simulink model "SiL_gram"  (R2025b)
settings: Solver=ode2  StartTime=0.0  StopTime=t_end  FixedStep=1/400  RelTol=1e-3
PreLoadFcn:
  | stepsize_sim = evalin('base', get_param(bdroot, 'FixedStep'));
undefined symbols (not defined in the file or in its folder): defaultConsts, defaultWP, DiscIntNeverNeededParam, dspblkCoreblockFVToolHelper, gcbh, navConsts, sensors, stepsize_ctrl
libraries: simulink x7, sharedutil x1, sharedtransform x1, aerolibanimutils x1
(part 1 of 3)
settings Model: Creator=ac112430  LastModifiedBy=ac124458
settings SolverCC: AlgebraicLoopSolver=TrustRegion
settings OptimizationCC: DefaultParameterBehavior=Inlined  DefaultUnderspecifiedDataType=single  ReuseModelBlockBuffer=off  PassReuseOutputArgsAs=Individual arguments  EfficientTunableParamExpr=on
settings DebuggingCC: ParameterPrecisionLossMsg=none  ParameterTunabilityLossMsg=error  UnconnectedInputMsg=warning  UnconnectedOutputMsg=warning  UnconnectedLineMsg=warning  ArithmeticOperatorsInVariantConditions=warning
settings HardwareCC: ProdBitPerPointer=32.0  ProdBitPerSizeT=32.0  ProdBitPerPtrDiffT=32.0  ProdLargestAtomicInteger=Long  ProdLargestAtomicFloat=Double  ProdIntDivRoundTo=Undefined  ProdWordSize=32.0  ProdHWDeviceType=ARM Compatible->ARM Cortex
settings ModelReferenceCC: EnableRefExpFcnMdlSchedulingChecks=on  ModelReferenceNumInstancesAllowed=Single  ModelReferenceMinAlgLoopOccurrences=on  PropagateSignalLabelsOutOfModel=off
settings SFSimCC: SimUseLocalCustomCode=off  MATLABDynamicMemAlloc=off  CustomCodeUndefinedFunction=UseInterfaceOnly
settings RTWCC: SystemTargetFile=ert.tlc  GenCodeOnly=on  TemplateMakefile=ert_default_tmf  RTWUseLocalCustomCode=off  IncludeHyperlinkInReport=on  GPUComputeCapability=3.5  Description=Embedded Coder
settings CodeAppCC: IgnoreCustomStorageClasses=off  StateflowObjectComments=on
settings ERTTargetCC: ERTCustomFileTemplate=example_file_process.tlc  ConvertIfToSwitch=off  SuppressUnreachableDefaultCases=off  DynamicArrayContainerType=coder::array  TargetLangStandard=C99 (ISO)  GenerateSampleERTMain=on  SupportComplex=off

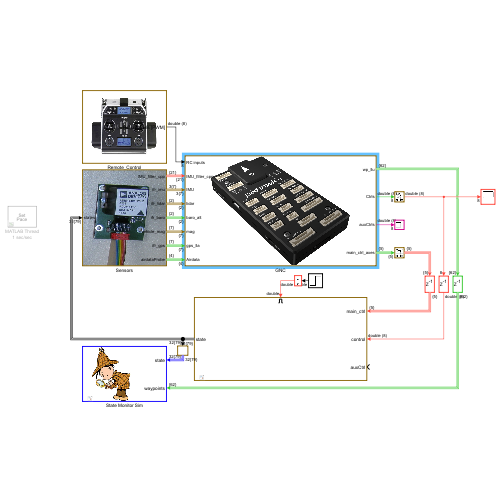
[thumbnail: Simulink's stored preview of the top-level diagram]
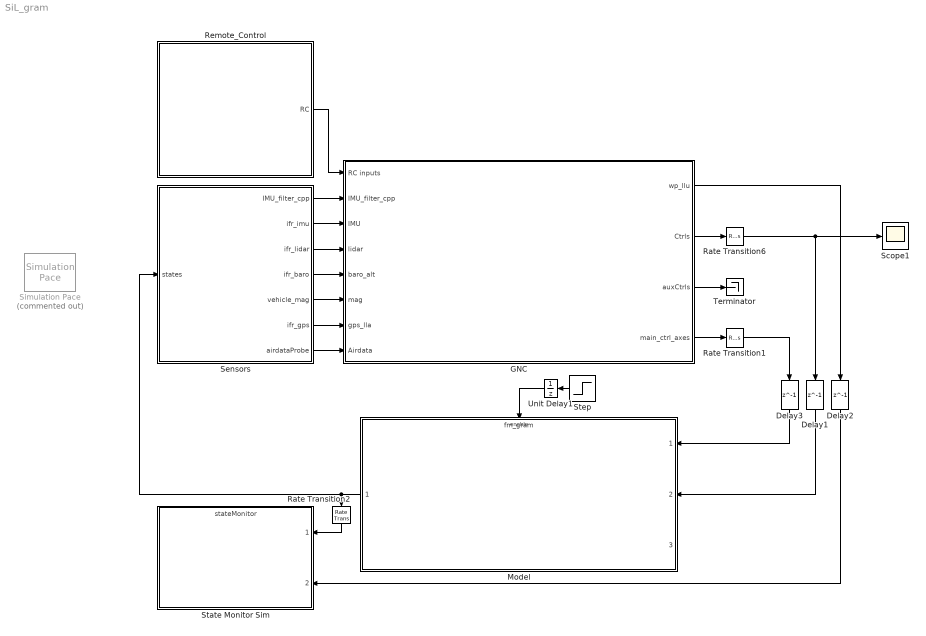
== system SiL_gram ==
  Delay1 : Delay  DelayLength=1  InitialCondition=0
  Delay2 : Delay  DelayLength=1  InitialCondition=0
  Delay3 : Delay  DelayLength=1  InitialCondition=0
  GNC : Subsystem
      mask Display:
      | image('figures/pixhawk2.png');
      | 
      | %port_label('input', 1, 'RC inputs');
      | %port_label('input', 2, 'IMU');
      | %port_label('input', 3, 'Optical Flow');
      | %port_label('input', 4, 'Sonar');
      | %port_label('input', 5, 'Barometer');
      | %port_label('input', 6, 'Magetometer');
      | %port_label('input', 7, 'GPS');
      | %port_label('input', 8, 'Airdata Probe');
      | 
      | %port_label('output', 1, 'Modes');
      | %port_label('output', 2, 'Warning ID');
      | %port_label('output', 3, 'State monitor data');
      | %port_label('output', 4, '(\delta \xi \eta \zeta \xi2 TW)^T', 'texmode', 'on');
      | %port_label('output', 5, 'Auxiliary controls', 'texmode', 'on');
      | %port_label('output', 6, '(x y z)_{ned}^T', 'texmode', 'on');
      | %port_label('output', 7, '(q1 q2 q3 q4)^T', 'texmode', 'on');
      | %port_label('output', 8, '(v_x v_y v_z)_{ned}^T', 'texmode', 'on');
      | %port_label('output', 9, '(v_{w,x} v_{w,y} v_{w,z})^T', 'texmode', 'on');
  Model : ModelReference  ModelNameDialog=fm_gram.slx  SimulationMode=Normal  ModelReferenceVersion=12.108  EnablePortName=Enable  EnablePortStatesWhenEnabling=held
      mask Display: %image('Library\figures\gram.jpg');
  Rate Transition1 : RateTransition  OutPortSampleTime=stepsize_sim
  Rate Transition2 : RateTransition  OutPortSampleTime=stepsize_mon
  Rate Transition6 : RateTransition  OutPortSampleTime=stepsize_sim
  Remote_Control : Subsystem
      mask Display:
      | image('figures/rc.png');
      | 
      | port_label('output', 1, 'RC channels [PWM]');
  Scope1 : Scope
      settings: ActiveDisplayYMinimum=-1.25  ActiveDisplayYMaximum=1.25
  Sensors : Subsystem
      mask Display:
      | image('figures/Sensoren.jpg');
      | 
      | %port_label('input', 1, 'State');
      | 
      | %port_label('output', 1, 'IMU');
      | %port_label('output', 2, 'Optical Flow');
      | %port_label('output', 3, 'Sonar');
      | %port_label('output', 4, 'Barometer');
      | %port_label('output', 5, 'Magnetometer');
      | %port_label('output', 6, 'GPS');
      | %port_label('output', 7, 'Airdata Probe');
  Simulation Pace : aerolibanimutils/Simulation Pace  Commented=on  SimulationPace=1  SleepMode=MATLAB Thread  OutputPaceError=off  SampleTime=-1
  State Monitor Sim : ModelReference  ModelNameDialog=stateMonitor.slx  SimulationMode=Normal  ModelReferenceVersion=12.19
      mask Display:
      | image('figures/detektiv2.png');
      | 
      | %port_label('input', 1, 'State');
      | %port_label('input', 2, 'V_{wind}','texmode','on');
      | %port_label('input', 3, 'State monitor data');
  Step : Step  Time=defaultConsts.forcesSuppressedTime  SampleTime=0
  Terminator : Terminator
  Unit Delay1 : UnitDelay  InitialCondition=1  SampleTime=-1  HasFrameUpgradeWarning=on
  wires:
  Sensors/2(ifr_imu) -> GNC/3(IMU)
  Sensors/3(ifr_lidar) -> GNC/4(lidar)
  Sensors/4(ifr_baro) -> GNC/5(baro_alt)
  Sensors/5(vehicle_mag) -> GNC/6(mag)
  Sensors/6(ifr_gps) -> GNC/7(gps_lla)
  Sensors/7(airdataProbe) -> GNC/8(Airdata)
  Remote_Control/1(RC) -> GNC/1(RC inputs)
  GNC/2(Ctrls) -> Rate Transition6/1
  GNC/1(wp_llu) -> Delay2/1
  Delay1/1 -> Model/2
  Model/1 -> Sensors/1(states), Rate Transition2/1
  Rate Transition2/1 -> State Monitor Sim/1
  Rate Transition6/1 -> Scope1/1, Delay1/1
  Sensors/1(IMU_filter_cpp) -> GNC/2(IMU_filter_cpp)
  Step/1 -> Unit Delay1/1
  Unit Delay1/1 -> Model/Enable
  Delay2/1 -> State Monitor Sim/2
  GNC/3(auxCtrls) -> Terminator/1
  GNC/4(main_ctrl_axes) -> Rate Transition1/1
  Delay3/1 -> Model/1
  Rate Transition1/1 -> Delay3/1

== system SiL_gram/GNC ==
  RC inputs : Inport
  IMU_filter_cpp : Inport  Port=2  OutDataTypeStr=Bus: ifr_imu_filtered_bus
  IMU : Inport  Port=3  OutDataTypeStr=Bus: ifr_imu
  lidar : Inport  Port=4  OutDataTypeStr=Bus: ifr_lidar
  baro_alt : Inport  Port=5  OutDataTypeStr=Bus: ifr_baro
  mag : Inport  Port=6  OutDataTypeStr=Bus: vehicle_magnetometer_bus
  gps_lla : Inport  Port=7  OutDataTypeStr=Bus: ifr_gps
  Airdata : Inport  Port=8  OutDataTypeStr=Bus: ifr_airdata
  EKF2_emulation : Subsystem
  Guidance_Control : Subsystem
  Postprocessing : Subsystem
  Unit Delay : UnitDelay  SampleTime=-1  HasFrameUpgradeWarning=on
  mavlink_receiver.cpp : Subsystem
  state_estimation : Subsystem
      settings: PortSchema="{\"entries\":[{\"content\":{\"sides\":[{\"content\":{\"connectorIds\":[\"In1\",\"In2\",\"In3\",\"In4\",\"In5\",\"In6\",\"In7\",\"In8\",\"In9\",\"In10\"]},\"type\":\"ConnectorPlacement.EquallySpacedRectSide\",\"uuid\":\"f704c686-db51-4285-959d-e889b94520cd\"},{\"content\":{\"connectorIds\":[\"Out1\",\"Out2\",\"Out3\",\"Out4\",\"Out5\",\"Out6\"],\"side\":\"RIGHT\"},\"type\":\"ConnectorPlacement.EquallySpacedRectSide\",\"uuid\":\"07b64360-9707-41f4-adee-da3792a52092\"},{\"content\":{\"connectorIds\":[\"In11\"],\"side\":\"TOP\"},\"type\":\"ConnectorPlacement.EquallySpacedRectSide\",\"uuid\":\"2f5e8d8a-3f45-40ad-b8f5-d38ec2cbea29\"}]},\"type\":\"ConnectorPlacement.EquallySpacedConnector\",\"uuid\":\"8dcdc60e-7634-4563-a6f8-beae9412036b\"}],\"packageUris\":[\"http://schema.mathworks.com/mf0/Connector/R2020b\"],\"version\":\"1.0\"}"
  wp_llu : Outport  OutDataTypeStr=Bus: waypoint_list_bus
  Ctrls : Outport  Port=2
  auxCtrls : Outport  Port=3
  main_ctrl_axes : Outport  Port=4  OutDataTypeStr=Bus: main_ctrl_axes_bus
  wires:
  Postprocessing/1(Ctrls) -> Ctrls/1
  RC inputs/1 -> mavlink_receiver.cpp/1(inputRC)
  IMU/1 -> mavlink_receiver.cpp/2(IMU)
  lidar/1 -> mavlink_receiver.cpp/3(lidar)
  baro_alt/1 -> mavlink_receiver.cpp/4(baro_alt)
  mag/1 -> mavlink_receiver.cpp/5(mag)
  gps_lla/1 -> mavlink_receiver.cpp/6(gps)
  Airdata/1 -> mavlink_receiver.cpp/7(Airdata)
  mavlink_receiver.cpp/9(RC channels) -> state_estimation/10(RC channels), Guidance_Control/12(RC channels)
  mavlink_receiver.cpp/1(Armed) -> state_estimation/2(armed)
  Guidance_Control/2(controls_0) -> Postprocessing/1(controls_0)
  mavlink_receiver.cpp/2(Time) -> state_estimation/3(clock)
  mavlink_receiver.cpp/3(Gyro) -> EKF2_emulation/2(gyro), state_estimation/4(gyro)
  mavlink_receiver.cpp/8(Accel) -> state_estimation/9(accel), EKF2_emulation/6(accel), Guidance_Control/11(sensor_accel)
  mavlink_receiver.cpp/4(baro) -> EKF2_emulation/3(baro), state_estimation/5(baro)
  mavlink_receiver.cpp/5(magmeter) -> EKF2_emulation/4(mag), state_estimation/6(mag)
  mavlink_receiver.cpp/6(gps_lla) -> EKF2_emulation/5(gps), state_estimation/7(gps)
  mavlink_receiver.cpp/7(status) -> state_estimation/8(status)
  state_estimation/1(time) -> Guidance_Control/2(clock)
  mavlink_receiver.cpp/10(waypoints) -> wp_llu/1, Guidance_Control/13(waypoint_list)
  Postprocessing/2(auxCtrls) -> auxCtrls/1
  Guidance_Control/3(controls_1) -> Postprocessing/2(controls_1)
  state_estimation/5(ac_state) -> Guidance_Control/6(ac_state)
  Unit Delay/1 -> state_estimation/11(main_ctrl_axes)
  state_estimation/3(act_limits) -> Guidance_Control/4(act_limits)
  state_estimation/2(RC_trim) -> Guidance_Control/3(RC_trim)
  state_estimation/4(track_deriv_moni) -> Guidance_Control/5(track_deriv_moni)
  IMU_filter_cpp/1 -> Guidance_Control/1(IMU_filter), EKF2_emulation/1(imu_filter), state_estimation/1(IMU_filter)
  state_estimation/6(RC_mode) -> Guidance_Control/7(RC_mode)
  Guidance_Control/1(main_ctrl_axes) -> main_ctrl_axes/1, Unit Delay/1
  EKF2_emulation/1(vehicle_local_position) -> Guidance_Control/8(vehicle_local_position)
  EKF2_emulation/2(vehicle_angular_velocity) -> Guidance_Control/9(vehicle_angular_velocity)
  EKF2_emulation/3(vehicle_attitude) -> Guidance_Control/10(vehicle_attitude)

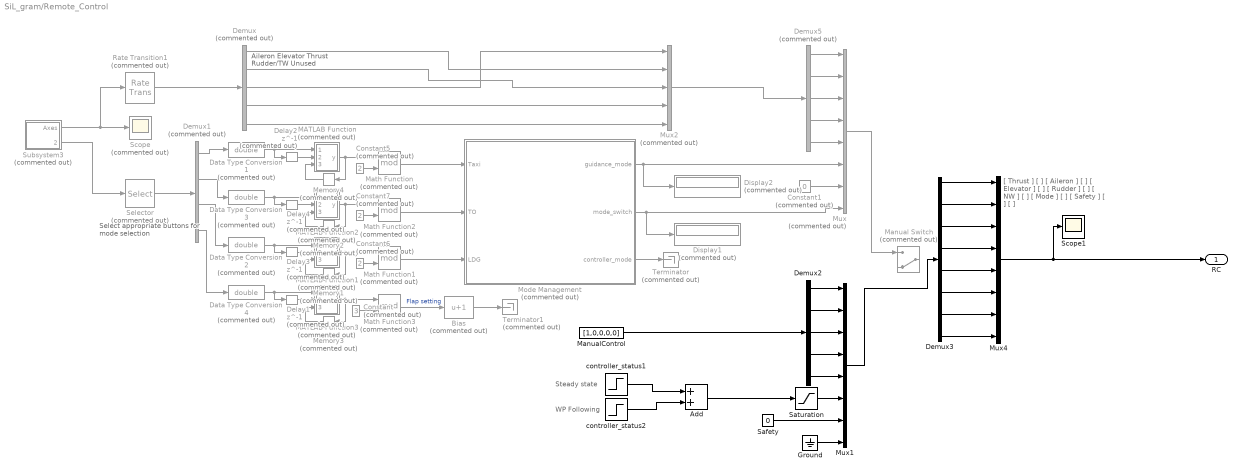
== system SiL_gram/Remote_Control ==
  note: Select appropriate
      | buttons for mode
      | selection
  note: Aileron
      |
      | Elevator
      |
      | Thrust
      |
      | Rudder/TW
      |
      | Unused
  note: [ Thrust ]
      | [ ]
      | [ Aileron ]
      | [ ]
      | [ Elevator ]
      | [ ]
      | [ Rudder ]
      | [ ]
      | [ NW ]
      | [ ]
      | [ Mode ]
      | [ ]
      | [ Safety ]
      | [ ]
      | [ ]
  note: Steady state
  note: WP Following
  Add : Sum
  Bias : Bias  Commented=on  Bias=1  SaturateOnIntegerOverflow=off
  Constant : Constant  Commented=on  Value=3  OutDataTypeStr=double
  Constant1 : Constant  Commented=on  Value=0
  Constant5 : Constant  Commented=on  Value=2
  Constant6 : Constant  Commented=on  Value=2
  Constant7 : Constant  Commented=on  Value=2
  Data Type Conversion{1..4} (4 alike) : DataTypeConversion  Commented=on  OutDataTypeStr=double  SaturateOnIntegerOverflow=off  RndMeth=Floor
  Delay{1..4} (4 alike) : Delay  Commented=on  DelayLength=1
  Demux : Demux  Commented=on  Outputs=5
  Demux1 : Demux  Commented=on
  Demux2 : Demux  Outputs=5
  Demux3 : Demux  Outputs=8
  Demux5 : Demux  Commented=on  Outputs=5
  Display1 : Display  Commented=on
  Display2 : Display  Commented=on
  Ground : Ground
  MATLAB Function : MATLAB Function  Commented=on  TreatAsAtomicUnit=on
  MATLAB Function1 : MATLAB Function  Commented=on  TreatAsAtomicUnit=on
  MATLAB Function2 : MATLAB Function  Commented=on  TreatAsAtomicUnit=on
  MATLAB Function3 : MATLAB Function  Commented=on  TreatAsAtomicUnit=on
  Manual Switch : ManualSwitch  Commented=on  CurrentSetting=0
  ManualControl : Constant  Value=[1,0,0,0,0]
  Math Function{,1..3} (4 alike) : Math  Commented=on  Operator=mod
  Memory1 : Memory  Commented=on  InheritSampleTime=on
  Memory2 : Memory  Commented=on  InheritSampleTime=on
  Memory3 : Memory  Commented=on  InheritSampleTime=on
  Memory4 : Memory  Commented=on  InheritSampleTime=on  LinearizeAsDelay=on
  "Mode Management " : Stateflow chart  Commented=on  TreatAsAtomicUnit=on
      settings: PortSchema="{\"entries\":[{\"content\":{\"sides\":[{\"content\":{\"connectorIds\":[\"In1\",\"In3\",\"In2\"]},\"type\":\"ConnectorPlacement.EquallySpacedRectSide\",\"uuid\":\"93057def-0b05-4e23-b054-e4bf056107a4\"},{\"content\":{\"connectorIds\":[\"Out2\",\"Out1\",\"Out3\"],\"side\":\"RIGHT\"},\"type\":\"ConnectorPlacement.EquallySpacedRectSide\",\"uuid\":\"acd3c48f-6b99-4bf7-86e8-be07c3648262\"},{\"content\":{\"connectorIds\":[],\"side\":\"TOP\"},\"type\":\"ConnectorPlacement.EquallySpacedRectSide\",\"uuid\":\"5e6f9e2e-3bd6-47db-ad7a-60b69db1e0b0\"}]},\"type\":\"ConnectorPlacement.EquallySpacedConnector\",\"uuid\":\"777f90d8-f88e-4555-b3e9-22ae8b9fb1af\"}],\"packageUris\":[\"http://schema.mathworks.com/mf0/Connector/19700101\"],\"version\":\"1.0\"}"
  Mux : Mux  Commented=on  Inputs=8
  Mux1 : Mux  Inputs=8
  Mux2 : Mux  Commented=on  Inputs=5
  Mux4 : Mux  Inputs=8
  Rate Transition1 : RateTransition  Commented=on  OutPortSampleTime=stepsize_sim
  Safety : Constant  Value=0
  Saturation : Saturate  UpperLimit=1  LowerLimit=-1
  Scope : Scope  Commented=on
      settings: ActiveDisplayYMinimum=-1.25  ActiveDisplayYMaximum=1.25
  Scope1 : Scope
      settings: ActiveDisplayYMinimum=-1.25  ActiveDisplayYMaximum=1.25
  Selector : Selector  Commented=on  InputPortWidth=12  IndexOptions=Index vector (dialog)  Indices=[5 6 7 9]  OutputSizes=1
  Subsystem3 : Subsystem  Commented=on
  Terminator : Terminator  Commented=on
  Terminator1 : Terminator  Commented=on
  controller_status1 : Step  Time=2  Before=-1  After=0  SampleTime=0
  controller_status2 : Step  Time=30  SampleTime=0
  RC : Outport  VectorParamsAs1DForOutWhenUnconnected=off
  wires:
  Demux/1 -> Mux2/2
  Rate Transition1/1 -> Demux/1
  Memory2/1 -> MATLAB Function2/3(val)
  Math Function/1 -> "Mode Management "/1(Taxi)
  Demux3/1 -> Mux4/1
  Demux/2 -> Mux2/3
  Delay3/1 -> MATLAB Function1/2(prev)
  Memory4/1 -> MATLAB Function/3(val)
  Data Type Conversion1/1 -> MATLAB Function/1(cur), Delay2/1
  Delay1/1 -> MATLAB Function3/2(prev)
  Bias/1 -> Terminator1/1
  "Mode Management "/1(mode_switch) -> Display1/1, Mux/8
  MATLAB Function1/1(y) -> Memory1/1, Math Function1/1
  Mux1/1 -> Demux3/1
  Demux1/2 -> Data Type Conversion3/1
  "Mode Management "/2(guidance_mode) -> Display2/1, Mux/6
  ManualControl/1 -> Demux2/1
  Demux1/4 -> Data Type Conversion4/1
  Demux/3 -> Mux2/1
  Demux1/1 -> Data Type Conversion1/1
  Subsystem3/2(Buttons) -> Selector/1
  Demux2/1 -> Mux1/1
  Delay2/1 -> MATLAB Function/2(prev)
  Memory1/1 -> MATLAB Function1/3(val)
  Demux3/8 -> Mux4/8
  MATLAB Function2/1(y) -> Math Function2/1, Memory2/1
  Demux3/2 -> Mux4/2
  Constant6/1 -> Math Function1/2
  Subsystem3/1(Axes) -> Rate Transition1/1, Scope/1
  Selector/1 -> Demux1/1
  Demux3/3 -> Mux4/3
  Data Type Conversion3/1 -> MATLAB Function2/1(cur), Delay4/1
  Math Function1/1 -> "Mode Management "/2(LDG)
  Demux3/7 -> Mux4/7
  Demux3/4 -> Mux4/4
  Demux5/1 -> Mux/1
  Demux/5 -> Mux2/5
  Mux2/1 -> Demux5/1
  MATLAB Function3/1(y) -> Math Function3/1, Memory3/1
  Data Type Conversion4/1 -> MATLAB Function3/1(cur), Delay1/1
  Safety/1 -> Mux1/7
  Mux/1 -> Manual Switch/1
  Demux5/2 -> Mux/2
  MATLAB Function/1(y) -> Math Function/1, Memory4/1
  Memory3/1 -> MATLAB Function3/3(val)
  Delay4/1 -> MATLAB Function2/2(prev)
  Demux3/6 -> Mux4/6
  Demux5/4 -> Mux/4
  Demux/4 -> Mux2/4
  Demux2/3 -> Mux1/3
  Math Function2/1 -> "Mode Management "/3(TO)
  Demux2/2 -> Mux1/2
  Constant7/1 -> Math Function2/2
  Demux2/4 -> Mux1/4
  Demux3/5 -> Mux4/5
  Math Function3/1 -> Bias/1  "Flap setting"
  Data Type Conversion2/1 -> Delay3/1, MATLAB Function1/1(cur)
  Demux1/3 -> Data Type Conversion2/1
  Demux2/5 -> Mux1/5
  Constant5/1 -> Math Function/2
  Demux5/5 -> Mux/5
  "Mode Management "/3(controller_mode) -> Terminator/1
  Demux5/3 -> Mux/3
  Constant1/1 -> Mux/7
  Constant/1 -> Math Function3/2
  Ground/1 -> Mux1/8
  Mux4/1 -> RC/1, Scope1/1
  controller_status2/1 -> Add/2
  controller_status1/1 -> Add/1
  Saturation/1 -> Mux1/6
  Add/1 -> Saturation/1

== system SiL_gram/Sensors ==
  states : Inport  OutDataTypeStr=Bus: fmBus
  Clock1 : Clock
  Data Type Conversion1 : DataTypeConversion  OutDataTypeStr=single  SaturateOnIntegerOverflow=off  RndMeth=Floor
  Fault_Simulation : Subsystem
  Rate Transition : RateTransition  OutPortSampleTime=stepsize_ctrl
  Rate Transition1 : RateTransition  OutPortSampleTime=stepsize_sim
  Sensor Model : ModelReference  ModelNameDialog=sensorModel.slx  SimulationMode=Normal  ModelReferenceVersion=12.17
  ifr_imu_filter.cpp : Subsystem
  IMU_filter_cpp : Outport  OutDataTypeStr=Bus: ifr_imu_filtered_bus
  ifr_imu : Outport  Port=2  OutDataTypeStr=Bus: ifr_imu  VectorParamsAs1DForOutWhenUnconnected=off
  ifr_lidar : Outport  Port=3  OutDataTypeStr=Bus: ifr_lidar  VectorParamsAs1DForOutWhenUnconnected=off
  ifr_baro : Outport  Port=4  OutDataTypeStr=Bus: ifr_baro  VectorParamsAs1DForOutWhenUnconnected=off
  vehicle_mag : Outport  Port=5  OutDataTypeStr=Bus: vehicle_magnetometer_bus  VectorParamsAs1DForOutWhenUnconnected=off
  ifr_gps : Outport  Port=6  OutDataTypeStr=Bus: ifr_gps  VectorParamsAs1DForOutWhenUnconnected=off
  airdataProbe : Outport  Port=7  OutDataTypeStr=Bus: ifr_airdata  VectorParamsAs1DForOutWhenUnconnected=off
  wires:
  Fault_Simulation/1(ifr_imu) -> ifr_imu/1
  Fault_Simulation/5(ifr_gps) -> ifr_gps/1
  Fault_Simulation/2(ifr_lidar) -> ifr_lidar/1
  Fault_Simulation/3(ifr_baro) -> ifr_baro/1
  Fault_Simulation/4(vehicle_mag) -> vehicle_mag/1
  Fault_Simulation/6(airdataProbe) -> airdataProbe/1
  Sensor Model/1 -> Rate Transition/1
  Clock1/1 -> Data Type Conversion1/1
  Data Type Conversion1/1 -> Fault_Simulation/1(time)
  states/1 -> Rate Transition1/1, Sensor Model/1
  ifr_imu_filter.cpp/1(IMU_filter) -> IMU_filter_cpp/1
  Rate Transition/1 -> Fault_Simulation/2(In1)
  Rate Transition1/1 -> ifr_imu_filter.cpp/1(state)

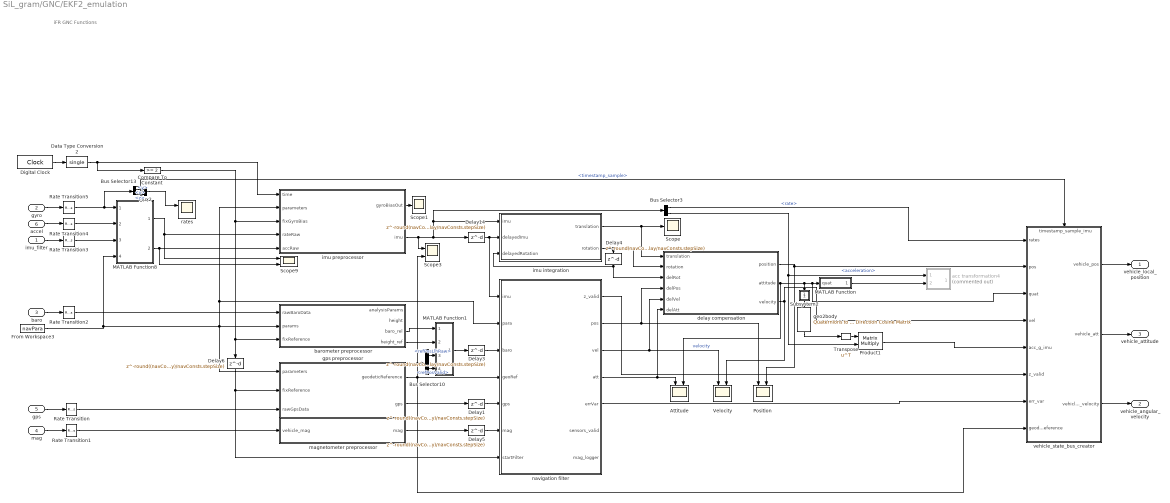
== system SiL_gram/GNC/EKF2_emulation ==
  note: iFR GNC Functions
  imu_filter : Inport  OutDataTypeStr=Bus: ifr_imu_filtered_bus
  gyro : Inport  Port=2  OutDataTypeStr=Bus: sensor_gyro_bus
  baro : Inport  Port=3  OutDataTypeStr=Bus: sensor_baro_bus
  mag : Inport  Port=4  OutDataTypeStr=Bus: vehicle_magnetometer_bus
  gps : Inport  Port=5  OutDataTypeStr=Bus: vehicle_gps_position_bus
  accel : Inport  Port=6  OutDataTypeStr=Bus: sensor_accel_bus
  Attitude : Scope  NumInputPorts=2
      settings: ActiveDisplayYMinimum=-1.23773  ActiveDisplayYMaximum=1.24864  DataLoggingVariableName=ScopeData11
  Bus Selector10 : BusSelector  OutputSignals=refPosLlhRaw,refPosValid
  Bus Selector13 : BusSelector  OutputSignals=timestamp_sample,x,y,z
  Bus Selector3 : BusSelector  OutputSignals=rate,acceleration
  Compare To Constant : simulink/Logic and Bit Operations/Compare To Constant  relop=>=  const=2  OutDataTypeStr=boolean
  Data Type Conversion2 : DataTypeConversion  OutDataTypeStr=single  SaturateOnIntegerOverflow=off  RndMeth=Floor
  Delay1 : Delay  DelayLength=round((navConsts.filterDelay-navConsts.gpsDelay)/navConsts.stepSize)  DelayLengthUpperLimit=300
  Delay14 : Delay  DelayLength=round(navConsts.filterDelay/navConsts.stepSize)  DelayLengthUpperLimit=300
  Delay3 : Delay  DelayLength=round(navConsts.filterDelay/navConsts.stepSize)  DelayLengthUpperLimit=300
  Delay4 : Delay  DelayLength=round(navConsts.filterDelay/navConsts.stepSize)  DelayLengthUpperLimit=300
  Delay5 : Delay  DelayLength=round((navConsts.filterDelay-navConsts.magDelay)/navConsts.stepSize)  DelayLengthUpperLimit=300
  Delay6 : Delay  DelayLength=round((navConsts.filterDelay-navConsts.magDelay)/navConsts.stepSize)  DelayLengthUpperLimit=300
  Digital Clock : DigitalClock  SampleTime=stepsize_ctrl
  From Workspace3 : FromWorkspace  VariableName=navPara  OutDataTypeStr=Bus: nav_parameterBus  SampleTime=stepsize_sim  Interpolate=off  OutputAfterFinalValue=Holding final value
  MATLAB Function : MATLAB Function  TreatAsAtomicUnit=on
  MATLAB Function1 : MATLAB Function  TreatAsAtomicUnit=on
  MATLAB Function8 : MATLAB Function  TreatAsAtomicUnit=on
  Mux2 : Mux  Inputs=3
  Position : Scope  NumInputPorts=2
      settings: ActiveDisplayYMinimum=-586.45755529403687  ActiveDisplayYMaximum=105.34517049789427  DataLoggingVariableName=ScopeData14
  Product1 : Product  Multiplication=Matrix(*)
  Rate Transition{,1..5} (6 alike) : RateTransition  OutPortSampleTime=stepsize_ctrl
  Scope : Scope
      settings: ActiveDisplayYMinimum=-1  ActiveDisplayYMaximum=1  DataLoggingVariableName=ScopeData5
  Scope1 : Scope
      settings: ActiveDisplayYMinimum=-0.099331239782016356  ActiveDisplayYMaximum=0.30195901907356948  DataLoggingVariableName=ScopeData15
  Scope3 : Scope  NumInputPorts=2
      settings: ActiveDisplayYMinimum=-0.2713911799557156  ActiveDisplayYMaximum=0.36740796754492377  DataLoggingVariableName=ScopeData16
  Scope9 : Scope  NumInputPorts=2
      settings: ActiveDisplayYMinimum=-1.8034829497337341  ActiveDisplayYMaximum=1.8379871249198914  DataLoggingVariableName=ScopeData13
  Subsystem2 : Subsystem
  Transpose : Math  Operator=transpose  SignedPower=on
  Velocity : Scope  NumInputPorts=2
      settings: ActiveDisplayYMinimum=-1  ActiveDisplayYMaximum=1  DataLoggingVariableName=ScopeData6
  acc transformation4 : MATLAB Function  Commented=on  TreatAsAtomicUnit=on
  barometer preprocessor : MATLAB Function  TreatAsAtomicUnit=on
  delay compensation : MATLAB Function  TreatAsAtomicUnit=on
  geo2body : sharedtransform/Quaternions to  Direction Cosine Matrix  aMode=aMode
  gps preprocessor : MATLAB Function  TreatAsAtomicUnit=on
  imu integration : MATLAB Function  TreatAsAtomicUnit=on
  imu preprocessor : MATLAB Function  TreatAsAtomicUnit=on
  magnetometer preprocessor : MATLAB Function  TreatAsAtomicUnit=on
  navigation filter : MATLAB Function  TreatAsAtomicUnit=on
  rates : Scope  NumInputPorts=2
      settings: ActiveDisplayYMinimum=-0.071955539506195931  ActiveDisplayYMaximum=0.11984543374486778  DataLoggingVariableName=ScopeData12
  vehicle_state_bus_creator : Subsystem
      settings: PortSchema="{\"entries\":[{\"content\":{\"sides\":[{\"content\":{\"connectorIds\":[\"In1\",\"In2\",\"In3\",\"In4\",\"In5\",\"In6\",\"In7\",\"In8\"]},\"type\":\"ConnectorPlacement.EquallySpacedRectSide\",\"uuid\":\"bc3ebfa1-daea-4709-952f-2fe4ea6771b8\"},{\"content\":{\"connectorIds\":[\"Out1\",\"Out2\",\"Out3\"],\"side\":\"RIGHT\"},\"type\":\"ConnectorPlacement.EquallySpacedRectSide\",\"uuid\":\"b99c6143-0656-4628-8455-051c6ced2792\"},{\"content\":{\"connectorIds\":[\"In9\"],\"side\":\"TOP\"},\"type\":\"ConnectorPlacement.EquallySpacedRectSide\",\"uuid\":\"81670970-0de5-4bc9-ac84-25aad24a7ec1\"},{\"content\":{\"side\":\"BOTTOM\"},\"type\":\"ConnectorPlacement.EquallySpacedRectSide\",\"uuid\":\"a3441f3b-1f80-4af6-b92c-bd0c79ef418a\"}]},\"type\":\"ConnectorPlacement.EquallySpacedConnector\",\"uuid\":\"3c725a23-f94b-421e-875e-8459dec9d453\"}],\"packageUris\":[\"http://schema.mathworks.com/mf0/Connector/R2020b\"],\"version\":\"1.0\"}"
  vehicle_local_position : Outport
  vehicle_angular_velocity : Outport  Port=2
  vehicle_attitude : Outport  Port=3
  wires:
  MATLAB Function8/2(acc_m) -> imu preprocessor/5(accRaw), Scope9/2
  barometer preprocessor/3(baro_rel) -> MATLAB Function1/1(baro_rel)
  Compare To Constant/1 -> Delay6/1, barometer preprocessor/3(fixReference), imu preprocessor/3(fixGyroBias)
  Bus Selector3/1 -> vehicle_state_bus_creator/1(rates)  "<rate>"
  MATLAB Function/1(eul_rad) -> acc transformation4/2(euler)
  gps preprocessor/1(geodeticReference) -> Scope3/2, Bus Selector10/1, vehicle_state_bus_creator/8(geodeticReference), navigation filter/4(geoRef)
  mag/1 -> Rate Transition1/1
  MATLAB Function8/1(gyro_m) -> Scope9/1, imu preprocessor/4(rateRaw)
  Delay1/1 -> navigation filter/5(gps)
  Delay4/1 -> delay compensation/3(delRot), imu integration/3(delayedRotation)
  navigation filter/4(att) -> delay compensation/6(delAtt), Attitude/1
  vehicle_state_bus_creator/2(vehicle_att) -> vehicle_attitude/1
  vehicle_state_bus_creator/3(vehicle_angular_velocity) -> vehicle_angular_velocity/1
  Delay6/1 -> navigation filter/7(startFilter), gps preprocessor/2(fixReference)
  navigation filter/5(errVar) -> vehicle_state_bus_creator/7(err_var)
  Delay14/1 -> imu integration/2(delayedImu), navigation filter/1(imu)
  Bus Selector13/2 -> Mux2/1  "<x>"
  delay compensation/3(velocity) -> vehicle_state_bus_creator/4(vel), Velocity/2
  MATLAB Function1/1(baro_abs) -> Delay3/1
  navigation filter/3(vel) -> Velocity/1, delay compensation/5(delVel)  "velocity"
  Bus Selector13/3 -> Mux2/2  "<y>"
  imu integration/2(rotation) -> delay compensation/2(rotation), Delay4/1
  Product1/1 -> vehicle_state_bus_creator/5(acc_g_imu)
  imu preprocessor/1(gyroBiasOut) -> Scope1/1
  imu integration/1(translation) -> Scope/1, delay compensation/1(translation)
  Delay5/1 -> navigation filter/6(mag)
  magnetometer preprocessor/1(mag) -> Delay5/1
  gps preprocessor/2(gps) -> Delay1/1
  accel/1 -> Rate Transition4/1
  baro/1 -> Rate Transition2/1
  Bus Selector10/1 -> MATLAB Function1/3(ref_pos)  "<refPosLlhRaw>"
  delay compensation/1(position) -> Position/2, vehicle_state_bus_creator/2(pos)
  vehicle_state_bus_creator/1(vehicle_pos) -> vehicle_local_position/1
  Bus Selector10/2 -> MATLAB Function1/4(ref_valid)  "<refPosValid>"
  Delay3/1 -> navigation filter/3(baro)
  gyro/1 -> Rate Transition5/1
  navigation filter/2(pos) -> Position/1, delay compensation/4(delPos)
  Bus Selector13/1 -> vehicle_state_bus_creator/9(timestamp_sample_imu)  "<timestamp_sample>"
  navigation filter/1(z_valid) -> vehicle_state_bus_creator/6(z_valid)
  Subsystem2/1(Out1) -> geo2body/1
  barometer preprocessor/4(height_ref) -> MATLAB Function1/2(h_ref)
  gps/1 -> Rate Transition/1
  From Workspace3/1 -> MATLAB Function8/4(param), imu preprocessor/2(parameters), navigation filter/2(para), gps preprocessor/1(parameters), barometer preprocessor/2(params)
  Bus Selector13/4 -> Mux2/3  "<z>"
  imu_filter/1 -> Rate Transition3/1
  Bus Selector3/2 -> acc transformation4/1(acc_b), Product1/2  "<acceleration>"
  imu preprocessor/2(imu) -> Bus Selector3/1, imu integration/1(imu), Delay14/1, Scope3/1
  Mux2/1 -> rates/1
  Digital Clock/1 -> Data Type Conversion2/1
  Data Type Conversion2/1 -> Compare To Constant/1, imu preprocessor/1(time)
  Rate Transition/1 -> gps preprocessor/3(rawGpsData)
  Rate Transition1/1 -> magnetometer preprocessor/1(vehicle_mag)
  Rate Transition2/1 -> barometer preprocessor/1(rawBaroData)
  Rate Transition3/1 -> MATLAB Function8/3(imu_filter)
  Rate Transition4/1 -> MATLAB Function8/2(acc_raw)
  Rate Transition5/1 -> Bus Selector13/1, MATLAB Function8/1(gyro_raw)
  geo2body/1 -> Transpose/1
  Transpose/1 -> Product1/1
  delay compensation/2(attitude) -> Attitude/2, vehicle_state_bus_creator/3(quat), MATLAB Function/1(quat), Subsystem2/1(" ")

== system SiL_gram/GNC/Guidance_Control ==
  IMU_filter : Inport  OutDataTypeStr=Bus: ifr_imu_filtered_bus
  clock : Inport  Port=2  OutDataTypeStr=single
  RC_trim : Inport  Port=3  OutDataTypeStr=Bus: rc_trim_bus
  act_limits : Inport  Port=4  OutDataTypeStr=Bus: actuator_limits_bus
  track_deriv_moni : Inport  Port=5  OutDataTypeStr=Bus: track_deriv_monitor_bus
  ac_state : Inport  Port=6  OutDataTypeStr=Bus: vehicle_state_bus
  RC_mode : Inport  Port=7  OutDataTypeStr=Bus: rc_mode_bus
  vehicle_local_position : Inport  Port=8  OutDataTypeStr=Bus: vehicle_local_position_bus
  vehicle_angular_velocity : Inport  Port=9  OutDataTypeStr=Bus: vehicle_angular_velocity_bus
  vehicle_attitude : Inport  Port=10  OutDataTypeStr=Bus: vehicle_attitude_bus
  sensor_accel : Inport  Port=11  OutDataTypeStr=Bus: sensor_accel_bus
  RC channels : Inport  Port=12  OutDataTypeStr=Bus: rc_channels_bus
  waypoint_list : Inport  Port=13  OutDataTypeStr=Bus: waypoint_list_bus
  From Workspace4 : FromWorkspace  VariableName=gncPara  OutDataTypeStr=Bus: gnc_parameterBus  SampleTime=stepsize_sim  Interpolate=off  OutputAfterFinalValue=Holding final value
  Terminator{,1..2,4,6} (5 alike) : Terminator
  atol_gnc : ModelReference  ModelNameDialog=gnc.slx  SimulationMode=Normal  ModelReferenceVersion=13.197
  main_ctrl_axes : Outport  OutDataTypeStr=Bus: main_ctrl_axes_bus
  controls_0 : Outport  Port=2  OutDataTypeStr=Bus: actuator_controls_0_bus  VectorParamsAs1DForOutWhenUnconnected=off
  controls_1 : Outport  Port=3  OutDataTypeStr=Bus: actuator_controls_1_bus  VectorParamsAs1DForOutWhenUnconnected=off
  wires:
  atol_gnc/1 -> Terminator1/1
  From Workspace4/1 -> atol_gnc/1
  atol_gnc/5 -> controls_1/1
  clock/1 -> atol_gnc/2
  atol_gnc/2 -> Terminator6/1
  atol_gnc/4 -> controls_0/1
  atol_gnc/3 -> Terminator4/1
  RC_mode/1 -> atol_gnc/9
  ac_state/1 -> atol_gnc/3
  act_limits/1 -> atol_gnc/4
  RC_trim/1 -> atol_gnc/5
  track_deriv_moni/1 -> atol_gnc/6
  IMU_filter/1 -> atol_gnc/7
  waypoint_list/1 -> atol_gnc/8
  atol_gnc/6 -> main_ctrl_axes/1
  vehicle_local_position/1 -> atol_gnc/10
  vehicle_angular_velocity/1 -> atol_gnc/11
  vehicle_attitude/1 -> atol_gnc/12
  sensor_accel/1 -> atol_gnc/14
  RC channels/1 -> atol_gnc/13
  atol_gnc/7 -> Terminator/1
  atol_gnc/8 -> Terminator2/1

== system SiL_gram/GNC/Postprocessing ==
  note: Align actuator signal sign to norm convention
  controls_0 : Inport  OutDataTypeStr=Bus: actuator_controls_0_bus
  controls_1 : Inport  Port=2  OutDataTypeStr=Bus: actuator_controls_0_bus
  Bus Selector1 : BusSelector  OutputSignals=control
  Bus Selector2 : BusSelector  OutputSignals=control
  Data Type Conversion2 : DataTypeConversion  OutDataTypeStr=double  SaturateOnIntegerOverflow=off  RndMeth=Floor
  Data Type Conversion4 : DataTypeConversion  OutDataTypeStr=double  SaturateOnIntegerOverflow=off  RndMeth=Floor
  Demux : Demux  Outputs=8
  Mux : Mux  Inputs=8
  Unary Minus : UnaryMinus  Commented=through
  Unary Minus1 : UnaryMinus  Commented=through
  Unary Minus2 : UnaryMinus  Commented=through
  Ctrls : Outport
  auxCtrls : Outport  Port=2
  wires:
  Data Type Conversion4/1 -> auxCtrls/1
  Data Type Conversion2/1 -> Ctrls/1
  controls_0/1 -> Bus Selector1/1
  controls_1/1 -> Bus Selector2/1
  Bus Selector2/1 -> Data Type Conversion4/1  "<control>"
  Bus Selector1/1 -> Demux/1  "<control>"
  Demux/8 -> Mux/8
  Demux/2 -> Unary Minus/1
  Demux/3 -> Unary Minus1/1
  Demux/4 -> Unary Minus2/1
  Demux/5 -> Mux/5
  Demux/6 -> Mux/6
  Demux/7 -> Mux/7
  Unary Minus/1 -> Mux/2
  Unary Minus1/1 -> Mux/3
  Demux/1 -> Mux/1
  Mux/1 -> Data Type Conversion2/1
  Unary Minus2/1 -> Mux/4

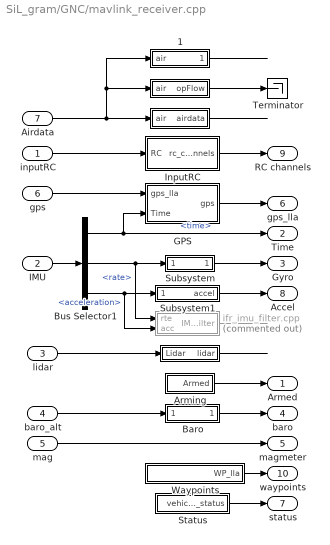
== system SiL_gram/GNC/mavlink_receiver.cpp ==
  inputRC : Inport
  IMU : Inport  Port=2  OutDataTypeStr=Bus: ifr_imu
  lidar : Inport  Port=3  OutDataTypeStr=Bus: ifr_lidar
  baro_alt : Inport  Port=4  OutDataTypeStr=Bus: ifr_baro
  mag : Inport  Port=5  OutDataTypeStr=Bus: vehicle_magnetometer_bus
  gps : Inport  Port=6  OutDataTypeStr=Bus: ifr_gps
  Airdata : Inport  Port=7  OutDataTypeStr=Bus: ifr_airdata
  " " : Subsystem
  "  " : Subsystem
  "   " : Subsystem
  " 1" : Subsystem
  Arming : Subsystem
  Baro : Subsystem
  Bus Selector1 : BusSelector  OutputSignals=time,rate,acceleration
  GPS : Subsystem
  InputRC : Subsystem
  Status : Subsystem
  Subsystem : Subsystem
  Subsystem1 : Subsystem
  Terminator : Terminator
  Waypoints : Subsystem
  ifr_imu_filter.cpp : Subsystem  Commented=on
  Armed : Outport  OutDataTypeStr=Bus: actuator_armed_bus
  Time : Outport  Port=2
  Gyro : Outport  Port=3  OutDataTypeStr=Bus: sensor_gyro_bus
  baro : Outport  Port=4  OutDataTypeStr=Bus: sensor_baro_bus
  magmeter : Outport  Port=5  OutDataTypeStr=Bus: vehicle_magnetometer_bus
  gps_lla : Outport  Port=6  OutDataTypeStr=Bus: vehicle_gps_position_bus
  status : Outport  Port=7  OutDataTypeStr=Bus: vehicle_status_bus
  Accel : Outport  Port=8  OutDataTypeStr=Bus: sensor_accel_bus
  RC channels : Outport  Port=9  OutDataTypeStr=Bus: rc_channels_bus
  waypoints : Outport  Port=10  OutDataTypeStr=Bus: waypoint_list_bus
  wires:
  lidar/1 -> "  "/1(Lidar)
  Arming/1(Armed) -> Armed/1
  InputRC/1(rc_channels) -> RC channels/1
  Baro/1(baro) -> baro/1
  inputRC/1 -> InputRC/1(RC)
  IMU/1 -> Bus Selector1/1
  GPS/1(gps) -> gps_lla/1
  baro_alt/1 -> Baro/1(p_alt)
  Bus Selector1/1 -> Time/1, GPS/2(Time)  "<time>"
  "   "/1(airdata) -> ?
  Subsystem1/1(accel) -> Accel/1
  gps/1 -> GPS/1(gps_lla)
  Bus Selector1/2 -> Subsystem/1(rate), ifr_imu_filter.cpp/1(rte)  "<rate>"
  Subsystem/1(Gyro) -> Gyro/1
  Bus Selector1/3 -> ifr_imu_filter.cpp/2(acc), Subsystem1/1(<accel>)  "<acceleration>"
  Waypoints/1(WP_lla) -> waypoints/1
  Status/1(vehicle_status) -> status/1
  "  "/1(lidar) -> ?
  " "/1(opFlow) -> Terminator/1
  Airdata/1 -> " 1"/1(air), " "/1(air), "   "/1(air)
  " 1"/1(adcReport) -> ?
  mag/1 -> magmeter/1
  ifr_imu_filter.cpp/1(IMU_filter) -> ?

== system SiL_gram/GNC/state_estimation ==
  note: (1) test_controls
      | (2) steady_state
      | (3) wp_tracking
  IMU_filter : Inport  OutDataTypeStr=Bus: ifr_imu_filtered_bus
  armed : Inport  Port=2  OutDataTypeStr=Bus: actuator_armed_bus
  clock : Inport  Port=3  OutDataTypeStr=single
  gyro : Inport  Port=4  OutDataTypeStr=Bus: sensor_gyro_bus
  baro : Inport  Port=5  OutDataTypeStr=Bus: sensor_baro_bus
  mag : Inport  Port=6  OutDataTypeStr=Bus: vehicle_magnetometer_bus
  gps : Inport  Port=7  OutDataTypeStr=Bus: vehicle_gps_position_bus
  status : Inport  Port=8  OutDataTypeStr=Bus: vehicle_status_bus  Interpolate=off  BusOutputAsStruct=on
  accel : Inport  Port=9  OutDataTypeStr=Bus: sensor_accel_bus
  RC channels : Inport  Port=10  OutDataTypeStr=Bus: rc_channels_bus
  main_ctrl_axes : Inport  Port=11  OutDataTypeStr=Bus: main_ctrl_axes_bus
  From Workspace3 : FromWorkspace  VariableName=navPara  OutDataTypeStr=Bus: nav_parameterBus  SampleTime=stepsize_sim  Interpolate=off  OutputAfterFinalValue=Holding final value
  Terminator{1..4} (4 alike) : Terminator
  state_estimation : ModelReference  ModelNameDialog=nav.slx  SimulationMode=Normal  ModelReferenceVersion=14.68
      settings: PortSchema="{\"entries\":[{\"content\":{\"sides\":[{\"content\":{\"connectorIds\":[\"In1\",\"In2\",\"In3\",\"In4\",\"In5\",\"In6\",\"In7\",\"In8\",\"In12\",\"In10\",\"In11\",\"In9\"]},\"type\":\"ConnectorPlacement.EquallySpacedRectSide\",\"uuid\":\"fd81afa0-68b0-4191-a2c5-81aa71d5f92f\"},{\"content\":{\"connectorIds\":[\"Out1\",\"Out2\",\"Out3\",\"Out4\",\"Out6\",\"Out5\",\"Out7\",\"Out8\",\"Out9\"],\"side\":\"RIGHT\"},\"type\":\"ConnectorPlacement.EquallySpacedRectSide\",\"uuid\":\"714f56d5-e6c0-4fef-84d4-d77db552ccd8\"},{\"content\":{\"side\":\"TOP\"},\"type\":\"ConnectorPlacement.EquallySpacedRectSide\",\"uuid\":\"18be0ae2-fd1a-4cc8-bcdc-2f29373e132e\"}]},\"type\":\"ConnectorPlacement.EquallySpacedConnector\",\"uuid\":\"f0e3624f-ec46-4046-8614-b93a2bfa50c6\"}],\"packageUris\":[\"http://schema.mathworks.com/mf0/Connector/R2020b\"],\"version\":\"1.0\"}"
  time : Outport
  RC_trim : Outport  Port=2  OutDataTypeStr=Bus: rc_trim_bus
  act_limits : Outport  Port=3  OutDataTypeStr=Bus: actuator_limits_bus
  track_deriv_moni : Outport  Port=4  OutDataTypeStr=Bus: track_deriv_monitor_bus
  ac_state : Outport  Port=5  OutDataTypeStr=Bus: vehicle_state_bus  VectorParamsAs1DForOutWhenUnconnected=off
  RC_mode : Outport  Port=6  OutDataTypeStr=Bus: rc_mode_bus
  wires:
  state_estimation/1 -> Terminator3/1
  state_estimation/4 -> Terminator2/1
  state_estimation/3 -> Terminator1/1
  state_estimation/2 -> Terminator4/1
  clock/1 -> time/1, state_estimation/1
  armed/1 -> state_estimation/2
  gyro/1 -> state_estimation/3
  accel/1 -> state_estimation/4
  baro/1 -> state_estimation/5
  mag/1 -> state_estimation/6
  state_estimation/5 -> ac_state/1
  state_estimation/6 -> RC_mode/1
  From Workspace3/1 -> state_estimation/9
  IMU_filter/1 -> state_estimation/11
  RC channels/1 -> state_estimation/10
  main_ctrl_axes/1 -> state_estimation/12
  gps/1 -> state_estimation/7
  status/1 -> state_estimation/8
  state_estimation/9 -> track_deriv_moni/1
  state_estimation/8 -> RC_trim/1
  state_estimation/7 -> act_limits/1

== system SiL_gram/Remote_Control/Subsystem3 ==
  note: After 2s:
      |   - Throttle from min to middle
      |   - Rudder/TW from neutral to +15%
  note: Throttle from min to max in 4 s
  note: All inputs in zero position
  note: Splineregler
  Constant : Constant  Value=2
  Constant1 : Constant  Value=[0 0 0 0 0 0 1 0 0 0 0 0]'
  Constant2 : Constant  Value=zeros(12,1)
  Manual Switch : ManualSwitch  CurrentSetting=0
  Multiport Switch : MultiPortSwitch  SaturateOnIntegerOverflow=off  InputSameDT=off
  Variant 1 : Subsystem
  Variant 2 : Subsystem
  Variant 3 : Subsystem
  Axes : Outport
  Buttons : Outport  Port=2
  wires:
  Constant2/1 -> Manual Switch/2
  Variant 3/1(Axes) -> Multiport Switch/4
  Constant/1 -> Multiport Switch/1
  Variant 2/1(Axes) -> Multiport Switch/3
  Variant 1/1(Axes) -> Multiport Switch/2
  Multiport Switch/1 -> Axes/1
  Constant1/1 -> Manual Switch/1
  Manual Switch/1 -> Buttons/1

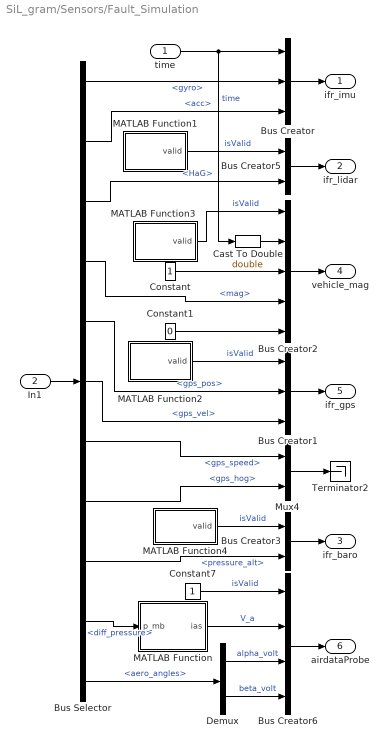
== system SiL_gram/Sensors/Fault_Simulation ==
  time : Inport
  In1 : Inport  Port=2  OutDataTypeStr=Bus: sensorBus
  Bus Creator : BusCreator  Inputs=3  OutDataTypeStr=Bus: ifr_imu
      settings: InheritFromInputs=off
  Bus Creator1 : BusCreator  Inputs=3  OutDataTypeStr=Bus: ifr_gps
      settings: InheritFromInputs=off
  Bus Creator2 : BusCreator  Inputs=5  OutDataTypeStr=Bus: vehicle_magnetometer_bus
      settings: InheritFromInputs=off
  Bus Creator3 : BusCreator  Inputs=2  OutDataTypeStr=Bus: ifr_baro
      settings: InheritFromInputs=off
  Bus Creator5 : BusCreator  Inputs=2  OutDataTypeStr=Bus: ifr_lidar
      settings: InheritFromInputs=off
  Bus Creator6 : BusCreator  Inputs=4
  Bus Selector : BusSelector  OutputSignals=gyro,acc,HaG,mag,gps_pos,gps_vel,gps_speed,gps_hog,pressure_alt,diff_pressure,aero_angles
  Cast To Double : DataTypeConversion  OutDataTypeStr=double  SaturateOnIntegerOverflow=off  RndMeth=Floor
  Constant : Constant  OutDataTypeStr=uint32
  Constant1 : Constant  Value=0  OutDataTypeStr=uint8
  Constant7 : Constant  OutDataTypeStr=boolean
  Demux : Demux  Outputs=2
  MATLAB Function : MATLAB Function  TreatAsAtomicUnit=on
  MATLAB Function1 : MATLAB Function  TreatAsAtomicUnit=on
  MATLAB Function2 : MATLAB Function  TreatAsAtomicUnit=on
  MATLAB Function3 : MATLAB Function  TreatAsAtomicUnit=on
  MATLAB Function4 : MATLAB Function  TreatAsAtomicUnit=on
  Mux4 : Mux  Inputs=2
  Terminator2 : Terminator
  ifr_imu : Outport  OutDataTypeStr=Bus: ifr_imu  VectorParamsAs1DForOutWhenUnconnected=off
  ifr_lidar : Outport  Port=2  OutDataTypeStr=Bus: ifr_lidar  VectorParamsAs1DForOutWhenUnconnected=off
  ifr_baro : Outport  Port=3  OutDataTypeStr=Bus: ifr_baro  VectorParamsAs1DForOutWhenUnconnected=off
  vehicle_mag : Outport  Port=4  OutDataTypeStr=Bus: vehicle_magnetometer_bus  VectorParamsAs1DForOutWhenUnconnected=off
  ifr_gps : Outport  Port=5  OutDataTypeStr=Bus: ifr_gps  VectorParamsAs1DForOutWhenUnconnected=off
  airdataProbe : Outport  Port=6  OutDataTypeStr=Bus: ifr_airdata  VectorParamsAs1DForOutWhenUnconnected=off
  wires:
  Bus Creator3/1 -> ifr_baro/1
  Bus Creator6/1 -> airdataProbe/1
  Bus Selector/5 -> Bus Creator1/2  "<gps_pos>"
  Bus Selector/2 -> Bus Creator/3  "<acc>"
  MATLAB Function2/1(valid) -> Bus Creator1/1  "isValid"
  Bus Creator1/1 -> ifr_gps/1
  Bus Creator2/1 -> vehicle_mag/1
  Bus Selector/1 -> Bus Creator/2  "<gyro>"
  time/1 -> Cast To Double/1, Bus Creator/1  "time"
  MATLAB Function1/1(valid) -> Bus Creator5/1  "isValid"
  Constant1/1 -> Bus Creator2/5
  Bus Selector/3 -> Bus Creator5/2  "<HaG>"
  Constant7/1 -> Bus Creator6/1  "isValid"
  Mux4/1 -> Terminator2/1
  Bus Selector/8 -> Mux4/2  "<gps_hog>"
  Constant/1 -> Bus Creator2/3
  Bus Selector/6 -> Bus Creator1/3  "<gps_vel>"
  MATLAB Function3/1(valid) -> Bus Creator2/1  "isValid"
  Bus Creator5/1 -> ifr_lidar/1
  Bus Selector/7 -> Mux4/1  "<gps_speed>"
  Bus Selector/10 -> MATLAB Function/1(p_mb)  "<diff_pressure>"
  MATLAB Function4/1(valid) -> Bus Creator3/1  "isValid"
  Demux/1 -> Bus Creator6/3  "alpha_volt"
  Bus Selector/4 -> Bus Creator2/4  "<mag>"
  Demux/2 -> Bus Creator6/4  "beta_volt"
  Bus Creator/1 -> ifr_imu/1
  Cast To Double/1 -> Bus Creator2/2
  In1/1 -> Bus Selector/1
  Bus Selector/9 -> Bus Creator3/2  "<pressure_alt>"
  MATLAB Function/1(ias) -> Bus Creator6/2  "V_a"
  Bus Selector/11 -> Demux/1  "<aero_angles>"

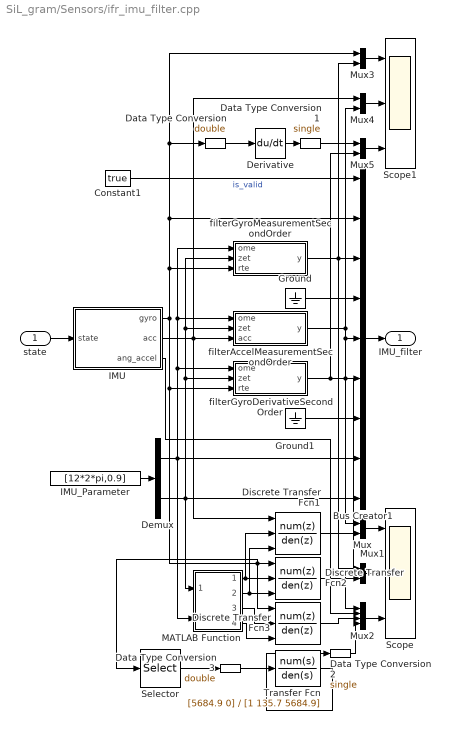
== system SiL_gram/Sensors/ifr_imu_filter.cpp ==
  state : Inport  OutDataTypeStr=Bus: fmBus
  Bus Creator1 : BusCreator  Inputs=9  OutDataTypeStr=Bus: ifr_imu_filtered_bus
      settings: InheritFromInputs=off
  Constant1 : Constant  Value=true  OutDataTypeStr=boolean
  Data Type Conversion : DataTypeConversion  OutDataTypeStr=double  SaturateOnIntegerOverflow=off  RndMeth=Floor
  Data Type Conversion1 : DataTypeConversion  OutDataTypeStr=single  SaturateOnIntegerOverflow=off  RndMeth=Floor
  Data Type Conversion2 : DataTypeConversion  OutDataTypeStr=single  SaturateOnIntegerOverflow=off  RndMeth=Floor
  Data Type Conversion3 : DataTypeConversion  OutDataTypeStr=double  SaturateOnIntegerOverflow=off  RndMeth=Floor
  Demux : Demux  Outputs=2
  Derivative : Derivative
  Discrete Transfer Fcn1 : DiscreteTransferFcn  NumeratorSource=Input port  DenominatorSource=Input port  a0EqualsOne=on
      settings: InputPortMap=u0,p1,p3
  Discrete Transfer Fcn2 : DiscreteTransferFcn  NumeratorSource=Input port  DenominatorSource=Input port  a0EqualsOne=on
      settings: InputPortMap=u0,p1,p3
  Discrete Transfer Fcn3 : DiscreteTransferFcn  LoadFcn=dspblkCoreblockFVToolHelper(gcbh,'load');  NumeratorSource=Input port  DenominatorSource=Input port  a0EqualsOne=on
      settings: CopyFcn=dspblkCoreblockFVToolHelper(gcbh,'copy');  DeleteFcn=dspblkCoreblockFVToolHelper(gcbh,'close');  ModelCloseFcn=dspblkCoreblockFVToolHelper(gcbh,'close');  PreSaveFcn=dspblkCoreblockFVToolHelper(gcbh,'presave');  PostSaveFcn=dspblkCoreblockFVToolHelper(gcbh,'postsave');  CloseFcn=dspblkCoreblockFVToolHelper(gcbh,'close');  InputPortMap=u0,p1,p3
  Ground : Ground
  Ground1 : Ground
  IMU : Subsystem
  IMU_Parameter : Constant  Value=[12*2*pi,0.9]  OutDataTypeStr=single
  MATLAB Function : MATLAB Function  TreatAsAtomicUnit=on
  Mux{,1,3..5} (5 alike) : Mux  Inputs=2
  Mux2 : Mux
  Scope : Scope  NumInputPorts=3
      settings: ActiveDisplayYMinimum=-34.5444992184639  ActiveDisplayYMaximum=9.3178895115852356  DataLoggingVariableName=ScopeData4
  Scope1 : Scope  NumInputPorts=3
      settings: ActiveDisplayYMinimum=-1.5383286625146866  ActiveDisplayYMaximum=1.5329927355051041
  Selector : Selector  InputPortWidth=3  IndexOptions=Index vector (dialog)  Indices=1  OutputSizes=1
  Transfer Fcn : TransferFcn  Numerator=[5684.9 0]  Denominator=[1 135.7 5684.9]
  filterAccelMeasurementSecondOrder : MATLAB Function  TreatAsAtomicUnit=on
  filterGyroDerivativeSecondOrder : MATLAB Function  TreatAsAtomicUnit=on
  filterGyroMeasurementSecondOrder : MATLAB Function  TreatAsAtomicUnit=on
  IMU_filter : Outport  OutDataTypeStr=Bus: ifr_imu_filtered_bus
  wires:
  Constant1/1 -> Bus Creator1/1  "is_valid"
  Bus Creator1/1 -> IMU_filter/1
  IMU_Parameter/1 -> Demux/1
  Demux/1 -> filterGyroDerivativeSecondOrder/1(ome), filterAccelMeasurementSecondOrder/1(ome), filterGyroMeasurementSecondOrder/1(ome), MATLAB Function/2(omega), Bus Creator1/8
  Demux/2 -> filterGyroDerivativeSecondOrder/2(zet), filterAccelMeasurementSecondOrder/2(zet), filterGyroMeasurementSecondOrder/2(zet), MATLAB Function/1(zeta), Bus Creator1/9
  IMU/2(acc) -> Mux4/1, Discrete Transfer Fcn1/1, filterAccelMeasurementSecondOrder/3(acc)
  IMU/1(gyro) -> Mux3/1, Data Type Conversion/1, Bus Creator1/2, filterGyroMeasurementSecondOrder/3(rte), Discrete Transfer Fcn3/1, Selector/1, Discrete Transfer Fcn2/1, filterGyroDerivativeSecondOrder/3(rte)
  filterGyroMeasurementSecondOrder/1(y) -> Mux1/1, Mux3/2, Bus Creator1/3
  Ground/1 -> Bus Creator1/4
  filterAccelMeasurementSecondOrder/1(y) -> Mux/1, Bus Creator1/5, Mux4/2
  filterGyroDerivativeSecondOrder/1(y) -> Bus Creator1/6, Mux2/1, Mux5/2
  Ground1/1 -> Bus Creator1/7
  MATLAB Function/4(diff_den) -> Discrete Transfer Fcn3/3
  MATLAB Function/3(diff_num) -> Discrete Transfer Fcn3/2
  MATLAB Function/2(filt_den) -> Discrete Transfer Fcn1/3, Discrete Transfer Fcn2/3
  MATLAB Function/1(filt_num) -> Discrete Transfer Fcn2/2, Discrete Transfer Fcn1/2
  Discrete Transfer Fcn1/1 -> Mux/2
  Discrete Transfer Fcn2/1 -> Mux1/2
  Discrete Transfer Fcn3/1 -> Mux2/3
  Mux1/1 -> Scope/2
  Mux2/1 -> Scope/3
  Mux/1 -> Scope/1
  Mux5/1 -> Scope1/3
  Mux4/1 -> Scope1/2
  Derivative/1 -> Data Type Conversion1/1
  Mux3/1 -> Scope1/1
  Data Type Conversion/1 -> Derivative/1
  Data Type Conversion1/1 -> Mux5/1
  state/1 -> IMU/1(state)
  IMU/3(ang_accel) -> Mux2/2
  Transfer Fcn/1 -> Data Type Conversion2/1
  Selector/1 -> Data Type Conversion3/1
  Data Type Conversion2/1 -> Mux2/4
  Data Type Conversion3/1 -> Transfer Fcn/1

== system SiL_gram/GNC/EKF2_emulation/Subsystem2 ==
  " " : Inport
  Compare To Constant : simulink/Logic and Bit Operations/Compare To Constant  relop===  const=0  OutDataTypeStr=boolean
  Constant : Constant  Value=[1;0;0;0]  OutDataTypeStr=single
  Quaternion Norm : sharedutil/Quaternion Norm  aMode=aMode
      settings: LibrarySourceBlock=|
      | aerolibutil/Quaternion
      | Norm
  Switch : Switch  Criteria=u2 > Threshold  SaturateOnIntegerOverflow=off  InputSameDT=off
  Out1 : Outport
  wires:
  " "/1 -> Switch/3, Quaternion Norm/1
  Quaternion Norm/1 -> Compare To Constant/1
  Compare To Constant/1 -> Switch/2
  Constant/1 -> Switch/1
  Switch/1 -> Out1/1
